simulink model "gm_ThreeSines_DrSaher"  (R2018a)
settings: Solver=FixedStepDiscrete  StartTime=0.0  StopTime=0.01  RelTol=1e-3
InitFcn:
  | ST = 2e-8
  | Ts = 2e-8
libraries: hdlmdlgenlib x97, hdlsllib x13, simulink x7, powerlib x1
(part 3 of 3)

== system gm_ThreeSines_DrSaher/Sines /cPA_Save ==
  MulNumber : Inport  PortDimensions=1  SampleTime=2e-08
  Enable : EnablePort
  MulResult : Outport  InitialOutput=0
  wires:
  MulNumber/1 -> MulResult/1

== system gm_ThreeSines_DrSaher/Sines /cPB_Save ==
  MulNumber : Inport  PortDimensions=1  SampleTime=2e-08
  Enable : EnablePort
  MulResult : Outport  InitialOutput=0
  wires:
  MulNumber/1 -> MulResult/1

== system gm_ThreeSines_DrSaher/Sines /cPC_Save ==
  MulNumber : Inport  PortDimensions=1  SampleTime=2e-08
  Enable : EnablePort
  MulResult : Outport  InitialOutput=0
  wires:
  MulNumber/1 -> MulResult/1

== system gm_ThreeSines_DrSaher/Sines /dPA_Save ==
  MulNumber : Inport  PortDimensions=1  SampleTime=2e-08
  Enable : EnablePort
  MulResult : Outport  InitialOutput=0
  wires:
  MulNumber/1 -> MulResult/1

== system gm_ThreeSines_DrSaher/Sines /dPB_Save ==
  MulNumber : Inport  PortDimensions=1  SampleTime=2e-08
  Enable : EnablePort
  MulResult : Outport  InitialOutput=0
  wires:
  MulNumber/1 -> MulResult/1

== system gm_ThreeSines_DrSaher/Sines /dPC_Save ==
  MulNumber : Inport  PortDimensions=1  SampleTime=2e-08
  Enable : EnablePort
  MulResult : Outport  InitialOutput=0
  wires:
  MulNumber/1 -> MulResult/1

== system gm_ThreeSines_DrSaher/Sines /HEX0/Subsystem ==
  Enable : EnablePort
  Constant9 : Constant  Value=64  OutMax=[64]  OutDataTypeStr=fixdt(0,7,0)  SampleTime=Ts
  0 : Outport  InitialOutput=0
  wires:
  Constant9/1 -> 0/1

== system gm_ThreeSines_DrSaher/Sines /HEX0/Subsystem10 ==
  Enable : EnablePort
  Constant9 : Constant  OutMax=[1]  OutDataTypeStr=fixdt(1,16,14)  SampleTime=Ts
  0 : Outport  InitialOutput=0
  wires:
  Constant9/1 -> 0/1

== system gm_ThreeSines_DrSaher/Sines /HEX0/Subsystem11 ==
  Enable : EnablePort
  Constant9 : Constant  Value=2  OutMax=[2]  OutDataTypeStr=fixdt(1,16,13)  SampleTime=Ts
  0 : Outport  InitialOutput=0
  wires:
  Constant9/1 -> 0/1

== system gm_ThreeSines_DrSaher/Sines /HEX0/Subsystem12 ==
  Enable : EnablePort
  Constant9 : Constant  Value=3  VectorParams1D=off  OutMax=[3]  OutDataTypeStr=fixdt(1,16,13)  SampleTime=Ts
  0 : Outport  InitialOutput=0
  wires:
  Constant9/1 -> 0/1

== system gm_ThreeSines_DrSaher/Sines /HEX0/Subsystem13 ==
  Enable : EnablePort
  Constant9 : Constant  Value=4  OutMax=[4]  OutDataTypeStr=fixdt(1,16,12)  SampleTime=Ts
  0 : Outport  InitialOutput=0
  wires:
  Constant9/1 -> 0/1

== system gm_ThreeSines_DrSaher/Sines /HEX0/Subsystem14 ==
  Enable : EnablePort
  Constant9 : Constant  Value=5  OutMax=[5]  OutDataTypeStr=fixdt(1,16,12)  SampleTime=Ts
  0 : Outport  InitialOutput=0
  wires:
  Constant9/1 -> 0/1

== system gm_ThreeSines_DrSaher/Sines /HEX0/Subsystem15 ==
  Enable : EnablePort
  Constant9 : Constant  Value=6  OutMax=[6]  OutDataTypeStr=fixdt(1,16,12)  SampleTime=Ts
  0 : Outport  InitialOutput=0
  wires:
  Constant9/1 -> 0/1

== system gm_ThreeSines_DrSaher/Sines /HEX0/Subsystem16 ==
  Enable : EnablePort
  Constant9 : Constant  Value=7  OutMax=[7]  OutDataTypeStr=fixdt(1,16,12)  SampleTime=Ts
  0 : Outport  InitialOutput=0
  wires:
  Constant9/1 -> 0/1

== system gm_ThreeSines_DrSaher/Sines /HEX0/Subsystem17 ==
  Enable : EnablePort
  Constant9 : Constant  Value=0  OutMax=[0]  OutDataTypeStr=fixdt(0,7,0)  SampleTime=Ts
  0 : Outport  InitialOutput=0
  wires:
  Constant9/1 -> 0/1

== system gm_ThreeSines_DrSaher/Sines /HEX0/Subsystem18 ==
  Enable : EnablePort
  Constant9 : Constant  Value=16  OutMax=[16]  OutDataTypeStr=fixdt(0,7,0)  SampleTime=Ts
  0 : Outport  InitialOutput=0
  wires:
  Constant9/1 -> 0/1

== system gm_ThreeSines_DrSaher/Sines /HEX0/Subsystem19 ==
  Enable : EnablePort
  Constant9 : Constant  Value=8  OutMax=[8]  OutDataTypeStr=fixdt(1,16,11)  SampleTime=Ts
  0 : Outport  InitialOutput=0
  wires:
  Constant9/1 -> 0/1

== system gm_ThreeSines_DrSaher/Sines /HEX0/Subsystem2 ==
  Enable : EnablePort
  Constant9 : Constant  Value=121  OutMax=[121]  OutDataTypeStr=fixdt(0,7,0)  SampleTime=Ts
  0 : Outport  InitialOutput=0
  wires:
  Constant9/1 -> 0/1

== system gm_ThreeSines_DrSaher/Sines /HEX0/Subsystem20 ==
  Enable : EnablePort
  Constant9 : Constant  Value=9  OutMax=[9]  OutDataTypeStr=fixdt(1,16,11)  SampleTime=Ts
  0 : Outport  InitialOutput=0
  wires:
  Constant9/1 -> 0/1

== system gm_ThreeSines_DrSaher/Sines /HEX0/Subsystem3 ==
  Enable : EnablePort
  Constant9 : Constant  Value=36  OutMax=[36]  OutDataTypeStr=fixdt(0,7,0)  SampleTime=Ts
  0 : Outport  InitialOutput=0
  wires:
  Constant9/1 -> 0/1

== system gm_ThreeSines_DrSaher/Sines /HEX0/Subsystem4 ==
  Enable : EnablePort
  Constant9 : Constant  Value=48  OutMax=[48]  OutDataTypeStr=fixdt(0,7,0)  SampleTime=Ts
  0 : Outport  InitialOutput=0
  wires:
  Constant9/1 -> 0/1

== system gm_ThreeSines_DrSaher/Sines /HEX0/Subsystem5 ==
  Enable : EnablePort
  Constant9 : Constant  Value=25  OutMax=[25]  OutDataTypeStr=fixdt(0,7,0)  SampleTime=Ts
  0 : Outport  InitialOutput=0
  wires:
  Constant9/1 -> 0/1

== system gm_ThreeSines_DrSaher/Sines /HEX0/Subsystem6 ==
  Enable : EnablePort
  Constant9 : Constant  Value=18  OutMax=[18]  OutDataTypeStr=fixdt(0,7,0)  SampleTime=Ts
  0 : Outport  InitialOutput=0
  wires:
  Constant9/1 -> 0/1

== system gm_ThreeSines_DrSaher/Sines /HEX0/Subsystem7 ==
  Enable : EnablePort
  Constant9 : Constant  Value=2  OutMax=[2]  OutDataTypeStr=fixdt(0,7,0)  SampleTime=Ts
  0 : Outport  InitialOutput=0
  wires:
  Constant9/1 -> 0/1

== system gm_ThreeSines_DrSaher/Sines /HEX0/Subsystem8 ==
  Enable : EnablePort
  Constant9 : Constant  Value=120  OutMax=[120]  OutDataTypeStr=fixdt(0,7,0)  SampleTime=Ts
  0 : Outport  InitialOutput=0
  wires:
  Constant9/1 -> 0/1

== system gm_ThreeSines_DrSaher/Sines /HEX0/Subsystem9 ==
  Enable : EnablePort
  Constant9 : Constant  Value=0  OutMax=[0]  OutDataTypeStr=fixdt(1,16,10)  SampleTime=Ts
  0 : Outport  InitialOutput=0
  wires:
  Constant9/1 -> 0/1

== system gm_ThreeSines_DrSaher/Sines /HEX1/Subsystem ==
  Enable : EnablePort
  Constant9 : Constant  Value=64  OutMax=[64]  OutDataTypeStr=fixdt(0,7,0)  SampleTime=Ts
  0 : Outport  InitialOutput=0
  wires:
  Constant9/1 -> 0/1

== system gm_ThreeSines_DrSaher/Sines /HEX1/Subsystem10 ==
  Enable : EnablePort
  Constant9 : Constant  OutMax=[1]  OutDataTypeStr=fixdt(1,16,14)  SampleTime=Ts
  0 : Outport  InitialOutput=0
  wires:
  Constant9/1 -> 0/1

== system gm_ThreeSines_DrSaher/Sines /HEX1/Subsystem11 ==
  Enable : EnablePort
  Constant9 : Constant  Value=2  OutMax=[2]  OutDataTypeStr=fixdt(1,16,13)  SampleTime=Ts
  0 : Outport  InitialOutput=0
  wires:
  Constant9/1 -> 0/1

== system gm_ThreeSines_DrSaher/Sines /HEX1/Subsystem12 ==
  Enable : EnablePort
  Constant9 : Constant  Value=3  VectorParams1D=off  OutMax=[3]  OutDataTypeStr=fixdt(1,16,13)  SampleTime=Ts
  0 : Outport  InitialOutput=0
  wires:
  Constant9/1 -> 0/1

== system gm_ThreeSines_DrSaher/Sines /HEX1/Subsystem13 ==
  Enable : EnablePort
  Constant9 : Constant  Value=4  OutMax=[4]  OutDataTypeStr=fixdt(1,16,12)  SampleTime=Ts
  0 : Outport  InitialOutput=0
  wires:
  Constant9/1 -> 0/1

== system gm_ThreeSines_DrSaher/Sines /HEX1/Subsystem14 ==
  Enable : EnablePort
  Constant9 : Constant  Value=5  OutMax=[5]  OutDataTypeStr=fixdt(1,16,12)  SampleTime=Ts
  0 : Outport  InitialOutput=0
  wires:
  Constant9/1 -> 0/1

== system gm_ThreeSines_DrSaher/Sines /HEX1/Subsystem15 ==
  Enable : EnablePort
  Constant9 : Constant  Value=6  OutMax=[6]  OutDataTypeStr=fixdt(1,16,12)  SampleTime=Ts
  0 : Outport  InitialOutput=0
  wires:
  Constant9/1 -> 0/1

== system gm_ThreeSines_DrSaher/Sines /HEX1/Subsystem16 ==
  Enable : EnablePort
  Constant9 : Constant  Value=7  OutMax=[7]  OutDataTypeStr=fixdt(1,16,12)  SampleTime=Ts
  0 : Outport  InitialOutput=0
  wires:
  Constant9/1 -> 0/1

== system gm_ThreeSines_DrSaher/Sines /HEX1/Subsystem17 ==
  Enable : EnablePort
  Constant9 : Constant  Value=0  OutMax=[0]  OutDataTypeStr=fixdt(0,7,0)  SampleTime=Ts
  0 : Outport  InitialOutput=0
  wires:
  Constant9/1 -> 0/1

== system gm_ThreeSines_DrSaher/Sines /HEX1/Subsystem18 ==
  Enable : EnablePort
  Constant9 : Constant  Value=16  OutMax=[16]  OutDataTypeStr=fixdt(0,7,0)  SampleTime=Ts
  0 : Outport  InitialOutput=0
  wires:
  Constant9/1 -> 0/1

== system gm_ThreeSines_DrSaher/Sines /HEX1/Subsystem19 ==
  Enable : EnablePort
  Constant9 : Constant  Value=8  OutMax=[8]  OutDataTypeStr=fixdt(1,16,11)  SampleTime=Ts
  0 : Outport  InitialOutput=0
  wires:
  Constant9/1 -> 0/1

== system gm_ThreeSines_DrSaher/Sines /HEX1/Subsystem2 ==
  Enable : EnablePort
  Constant9 : Constant  Value=121  OutMax=[121]  OutDataTypeStr=fixdt(0,7,0)  SampleTime=Ts
  0 : Outport  InitialOutput=0
  wires:
  Constant9/1 -> 0/1

== system gm_ThreeSines_DrSaher/Sines /HEX1/Subsystem20 ==
  Enable : EnablePort
  Constant9 : Constant  Value=9  OutMax=[9]  OutDataTypeStr=fixdt(1,16,11)  SampleTime=Ts
  0 : Outport  InitialOutput=0
  wires:
  Constant9/1 -> 0/1

== system gm_ThreeSines_DrSaher/Sines /HEX1/Subsystem3 ==
  Enable : EnablePort
  Constant9 : Constant  Value=36  OutMax=[36]  OutDataTypeStr=fixdt(0,7,0)  SampleTime=Ts
  0 : Outport  InitialOutput=0
  wires:
  Constant9/1 -> 0/1

== system gm_ThreeSines_DrSaher/Sines /HEX1/Subsystem4 ==
  Enable : EnablePort
  Constant9 : Constant  Value=48  OutMax=[48]  OutDataTypeStr=fixdt(0,7,0)  SampleTime=Ts
  0 : Outport  InitialOutput=0
  wires:
  Constant9/1 -> 0/1

== system gm_ThreeSines_DrSaher/Sines /HEX1/Subsystem5 ==
  Enable : EnablePort
  Constant9 : Constant  Value=25  OutMax=[25]  OutDataTypeStr=fixdt(0,7,0)  SampleTime=Ts
  0 : Outport  InitialOutput=0
  wires:
  Constant9/1 -> 0/1

== system gm_ThreeSines_DrSaher/Sines /HEX1/Subsystem6 ==
  Enable : EnablePort
  Constant9 : Constant  Value=18  OutMax=[18]  OutDataTypeStr=fixdt(0,7,0)  SampleTime=Ts
  0 : Outport  InitialOutput=0
  wires:
  Constant9/1 -> 0/1

== system gm_ThreeSines_DrSaher/Sines /HEX1/Subsystem7 ==
  Enable : EnablePort
  Constant9 : Constant  Value=2  OutMax=[2]  OutDataTypeStr=fixdt(0,7,0)  SampleTime=Ts
  0 : Outport  InitialOutput=0
  wires:
  Constant9/1 -> 0/1

== system gm_ThreeSines_DrSaher/Sines /HEX1/Subsystem8 ==
  Enable : EnablePort
  Constant9 : Constant  Value=120  OutMax=[120]  OutDataTypeStr=fixdt(0,7,0)  SampleTime=Ts
  0 : Outport  InitialOutput=0
  wires:
  Constant9/1 -> 0/1

== system gm_ThreeSines_DrSaher/Sines /HEX1/Subsystem9 ==
  Enable : EnablePort
  Constant9 : Constant  Value=0  OutMax=[0]  OutDataTypeStr=fixdt(1,16,10)  SampleTime=Ts
  0 : Outport  InitialOutput=0
  wires:
  Constant9/1 -> 0/1

== system gm_ThreeSines_DrSaher/Sines /HEX2/Subsystem ==
  Enable : EnablePort
  Constant9 : Constant  Value=64  OutMax=[64]  OutDataTypeStr=fixdt(0,7,0)  SampleTime=Ts
  0 : Outport  InitialOutput=0
  wires:
  Constant9/1 -> 0/1

== system gm_ThreeSines_DrSaher/Sines /HEX2/Subsystem10 ==
  Enable : EnablePort
  Constant9 : Constant  OutMax=[1]  OutDataTypeStr=fixdt(1,16,14)  SampleTime=Ts
  0 : Outport  InitialOutput=0
  wires:
  Constant9/1 -> 0/1

== system gm_ThreeSines_DrSaher/Sines /HEX2/Subsystem11 ==
  Enable : EnablePort
  Constant9 : Constant  Value=2  OutMax=[2]  OutDataTypeStr=fixdt(1,16,13)  SampleTime=Ts
  0 : Outport  InitialOutput=0
  wires:
  Constant9/1 -> 0/1

== system gm_ThreeSines_DrSaher/Sines /HEX2/Subsystem12 ==
  Enable : EnablePort
  Constant9 : Constant  Value=3  VectorParams1D=off  OutMax=[3]  OutDataTypeStr=fixdt(1,16,13)  SampleTime=Ts
  0 : Outport  InitialOutput=0
  wires:
  Constant9/1 -> 0/1

== system gm_ThreeSines_DrSaher/Sines /HEX2/Subsystem13 ==
  Enable : EnablePort
  Constant9 : Constant  Value=4  OutMax=[4]  OutDataTypeStr=fixdt(1,16,12)  SampleTime=Ts
  0 : Outport  InitialOutput=0
  wires:
  Constant9/1 -> 0/1

== system gm_ThreeSines_DrSaher/Sines /HEX2/Subsystem14 ==
  Enable : EnablePort
  Constant9 : Constant  Value=5  OutMax=[5]  OutDataTypeStr=fixdt(1,16,12)  SampleTime=Ts
  0 : Outport  InitialOutput=0
  wires:
  Constant9/1 -> 0/1

== system gm_ThreeSines_DrSaher/Sines /HEX2/Subsystem15 ==
  Enable : EnablePort
  Constant9 : Constant  Value=6  OutMax=[6]  OutDataTypeStr=fixdt(1,16,12)  SampleTime=Ts
  0 : Outport  InitialOutput=0
  wires:
  Constant9/1 -> 0/1

== system gm_ThreeSines_DrSaher/Sines /HEX2/Subsystem16 ==
  Enable : EnablePort
  Constant9 : Constant  Value=7  OutMax=[7]  OutDataTypeStr=fixdt(1,16,12)  SampleTime=Ts
  0 : Outport  InitialOutput=0
  wires:
  Constant9/1 -> 0/1

== system gm_ThreeSines_DrSaher/Sines /HEX2/Subsystem17 ==
  Enable : EnablePort
  Constant9 : Constant  Value=0  OutMax=[0]  OutDataTypeStr=fixdt(0,7,0)  SampleTime=Ts
  0 : Outport  InitialOutput=0
  wires:
  Constant9/1 -> 0/1

== system gm_ThreeSines_DrSaher/Sines /HEX2/Subsystem18 ==
  Enable : EnablePort
  Constant9 : Constant  Value=16  OutMax=[16]  OutDataTypeStr=fixdt(0,7,0)  SampleTime=Ts
  0 : Outport  InitialOutput=0
  wires:
  Constant9/1 -> 0/1

== system gm_ThreeSines_DrSaher/Sines /HEX2/Subsystem19 ==
  Enable : EnablePort
  Constant9 : Constant  Value=8  OutMax=[8]  OutDataTypeStr=fixdt(1,16,11)  SampleTime=Ts
  0 : Outport  InitialOutput=0
  wires:
  Constant9/1 -> 0/1

== system gm_ThreeSines_DrSaher/Sines /HEX2/Subsystem2 ==
  Enable : EnablePort
  Constant9 : Constant  Value=121  OutMax=[121]  OutDataTypeStr=fixdt(0,7,0)  SampleTime=Ts
  0 : Outport  InitialOutput=0
  wires:
  Constant9/1 -> 0/1

== system gm_ThreeSines_DrSaher/Sines /HEX2/Subsystem20 ==
  Enable : EnablePort
  Constant9 : Constant  Value=9  OutMax=[9]  OutDataTypeStr=fixdt(1,16,11)  SampleTime=Ts
  0 : Outport  InitialOutput=0
  wires:
  Constant9/1 -> 0/1

== system gm_ThreeSines_DrSaher/Sines /HEX2/Subsystem3 ==
  Enable : EnablePort
  Constant9 : Constant  Value=36  OutMax=[36]  OutDataTypeStr=fixdt(0,7,0)  SampleTime=Ts
  0 : Outport  InitialOutput=0
  wires:
  Constant9/1 -> 0/1

== system gm_ThreeSines_DrSaher/Sines /HEX2/Subsystem4 ==
  Enable : EnablePort
  Constant9 : Constant  Value=48  OutMax=[48]  OutDataTypeStr=fixdt(0,7,0)  SampleTime=Ts
  0 : Outport  InitialOutput=0
  wires:
  Constant9/1 -> 0/1

== system gm_ThreeSines_DrSaher/Sines /HEX2/Subsystem5 ==
  Enable : EnablePort
  Constant9 : Constant  Value=25  OutMax=[25]  OutDataTypeStr=fixdt(0,7,0)  SampleTime=Ts
  0 : Outport  InitialOutput=0
  wires:
  Constant9/1 -> 0/1

== system gm_ThreeSines_DrSaher/Sines /HEX2/Subsystem6 ==
  Enable : EnablePort
  Constant9 : Constant  Value=18  OutMax=[18]  OutDataTypeStr=fixdt(0,7,0)  SampleTime=Ts
  0 : Outport  InitialOutput=0
  wires:
  Constant9/1 -> 0/1

== system gm_ThreeSines_DrSaher/Sines /HEX2/Subsystem7 ==
  Enable : EnablePort
  Constant9 : Constant  Value=2  OutMax=[2]  OutDataTypeStr=fixdt(0,7,0)  SampleTime=Ts
  0 : Outport  InitialOutput=0
  wires:
  Constant9/1 -> 0/1

== system gm_ThreeSines_DrSaher/Sines /HEX2/Subsystem8 ==
  Enable : EnablePort
  Constant9 : Constant  Value=120  OutMax=[120]  OutDataTypeStr=fixdt(0,7,0)  SampleTime=Ts
  0 : Outport  InitialOutput=0
  wires:
  Constant9/1 -> 0/1

== system gm_ThreeSines_DrSaher/Sines /HEX2/Subsystem9 ==
  Enable : EnablePort
  Constant9 : Constant  Value=0  OutMax=[0]  OutDataTypeStr=fixdt(1,16,10)  SampleTime=Ts
  0 : Outport  InitialOutput=0
  wires:
  Constant9/1 -> 0/1

== system gm_ThreeSines_DrSaher/Sines /HEX3/Subsystem ==
  Enable : EnablePort
  Constant9 : Constant  Value=64  OutMax=[64]  OutDataTypeStr=fixdt(0,7,0)  SampleTime=Ts
  0 : Outport  InitialOutput=0
  wires:
  Constant9/1 -> 0/1

== system gm_ThreeSines_DrSaher/Sines /HEX3/Subsystem10 ==
  Enable : EnablePort
  Constant9 : Constant  OutMax=[1]  OutDataTypeStr=fixdt(1,16,14)  SampleTime=Ts
  0 : Outport  InitialOutput=0
  wires:
  Constant9/1 -> 0/1

== system gm_ThreeSines_DrSaher/Sines /HEX3/Subsystem11 ==
  Enable : EnablePort
  Constant9 : Constant  Value=2  OutMax=[2]  OutDataTypeStr=fixdt(1,16,13)  SampleTime=Ts
  0 : Outport  InitialOutput=0
  wires:
  Constant9/1 -> 0/1

== system gm_ThreeSines_DrSaher/Sines /HEX3/Subsystem12 ==
  Enable : EnablePort
  Constant9 : Constant  Value=3  VectorParams1D=off  OutMax=[3]  OutDataTypeStr=fixdt(1,16,13)  SampleTime=Ts
  0 : Outport  InitialOutput=0
  wires:
  Constant9/1 -> 0/1

== system gm_ThreeSines_DrSaher/Sines /HEX3/Subsystem13 ==
  Enable : EnablePort
  Constant9 : Constant  Value=4  OutMax=[4]  OutDataTypeStr=fixdt(1,16,12)  SampleTime=Ts
  0 : Outport  InitialOutput=0
  wires:
  Constant9/1 -> 0/1

== system gm_ThreeSines_DrSaher/Sines /HEX3/Subsystem14 ==
  Enable : EnablePort
  Constant9 : Constant  Value=5  OutMax=[5]  OutDataTypeStr=fixdt(1,16,12)  SampleTime=Ts
  0 : Outport  InitialOutput=0
  wires:
  Constant9/1 -> 0/1

== system gm_ThreeSines_DrSaher/Sines /HEX3/Subsystem15 ==
  Enable : EnablePort
  Constant9 : Constant  Value=6  OutMax=[6]  OutDataTypeStr=fixdt(1,16,12)  SampleTime=Ts
  0 : Outport  InitialOutput=0
  wires:
  Constant9/1 -> 0/1

== system gm_ThreeSines_DrSaher/Sines /HEX3/Subsystem16 ==
  Enable : EnablePort
  Constant9 : Constant  Value=7  OutMax=[7]  OutDataTypeStr=fixdt(1,16,12)  SampleTime=Ts
  0 : Outport  InitialOutput=0
  wires:
  Constant9/1 -> 0/1

== system gm_ThreeSines_DrSaher/Sines /HEX3/Subsystem17 ==
  Enable : EnablePort
  Constant9 : Constant  Value=0  OutMax=[0]  OutDataTypeStr=fixdt(0,7,0)  SampleTime=Ts
  0 : Outport  InitialOutput=0
  wires:
  Constant9/1 -> 0/1

== system gm_ThreeSines_DrSaher/Sines /HEX3/Subsystem18 ==
  Enable : EnablePort
  Constant9 : Constant  Value=16  OutMax=[16]  OutDataTypeStr=fixdt(0,7,0)  SampleTime=Ts
  0 : Outport  InitialOutput=0
  wires:
  Constant9/1 -> 0/1

== system gm_ThreeSines_DrSaher/Sines /HEX3/Subsystem19 ==
  Enable : EnablePort
  Constant9 : Constant  Value=8  OutMax=[8]  OutDataTypeStr=fixdt(1,16,11)  SampleTime=Ts
  0 : Outport  InitialOutput=0
  wires:
  Constant9/1 -> 0/1

== system gm_ThreeSines_DrSaher/Sines /HEX3/Subsystem2 ==
  Enable : EnablePort
  Constant9 : Constant  Value=121  OutMax=[121]  OutDataTypeStr=fixdt(0,7,0)  SampleTime=Ts
  0 : Outport  InitialOutput=0
  wires:
  Constant9/1 -> 0/1

== system gm_ThreeSines_DrSaher/Sines /HEX3/Subsystem20 ==
  Enable : EnablePort
  Constant9 : Constant  Value=9  OutMax=[9]  OutDataTypeStr=fixdt(1,16,11)  SampleTime=Ts
  0 : Outport  InitialOutput=0
  wires:
  Constant9/1 -> 0/1

== system gm_ThreeSines_DrSaher/Sines /HEX3/Subsystem3 ==
  Enable : EnablePort
  Constant9 : Constant  Value=36  OutMax=[36]  OutDataTypeStr=fixdt(0,7,0)  SampleTime=Ts
  0 : Outport  InitialOutput=0
  wires:
  Constant9/1 -> 0/1

== system gm_ThreeSines_DrSaher/Sines /HEX3/Subsystem4 ==
  Enable : EnablePort
  Constant9 : Constant  Value=48  OutMax=[48]  OutDataTypeStr=fixdt(0,7,0)  SampleTime=Ts
  0 : Outport  InitialOutput=0
  wires:
  Constant9/1 -> 0/1

== system gm_ThreeSines_DrSaher/Sines /HEX3/Subsystem5 ==
  Enable : EnablePort
  Constant9 : Constant  Value=25  OutMax=[25]  OutDataTypeStr=fixdt(0,7,0)  SampleTime=Ts
  0 : Outport  InitialOutput=0
  wires:
  Constant9/1 -> 0/1

== system gm_ThreeSines_DrSaher/Sines /HEX3/Subsystem6 ==
  Enable : EnablePort
  Constant9 : Constant  Value=18  OutMax=[18]  OutDataTypeStr=fixdt(0,7,0)  SampleTime=Ts
  0 : Outport  InitialOutput=0
  wires:
  Constant9/1 -> 0/1

== system gm_ThreeSines_DrSaher/Sines /HEX3/Subsystem7 ==
  Enable : EnablePort
  Constant9 : Constant  Value=2  OutMax=[2]  OutDataTypeStr=fixdt(0,7,0)  SampleTime=Ts
  0 : Outport  InitialOutput=0
  wires:
  Constant9/1 -> 0/1

== system gm_ThreeSines_DrSaher/Sines /HEX3/Subsystem8 ==
  Enable : EnablePort
  Constant9 : Constant  Value=120  OutMax=[120]  OutDataTypeStr=fixdt(0,7,0)  SampleTime=Ts
  0 : Outport  InitialOutput=0
  wires:
  Constant9/1 -> 0/1

== system gm_ThreeSines_DrSaher/Sines /HEX3/Subsystem9 ==
  Enable : EnablePort
  Constant9 : Constant  Value=0  OutMax=[0]  OutDataTypeStr=fixdt(1,16,10)  SampleTime=Ts
  0 : Outport  InitialOutput=0
  wires:
  Constant9/1 -> 0/1
